simulink model "pid_pos"  (R2021a)
settings: Solver=ode5  StartTime=0.0  StopTime=15  MaxStep=0.001  RelTol=1e-3  EnableMultiTasking=on
values from neighbouring files (symbols this model uses):
  Kd = 0.158    [my_real_pendulum.m]
  Kd_phi = 0.22    [my_real_pendulum.m]
  Ki = 0.136    [my_real_pendulum.m]
  Kp = 0.522    [my_real_pendulum.m]
undefined symbols (not defined in the file or in its folder): Humusoft, MF624
libraries: sldrtlib x3, slpidlib x2, simulink x2
settings Model: Creator=fuka  LastModifiedBy=koubajac
settings SolverCC: AlgebraicLoopSolver=TrustRegion
settings DataIOCC: LimitDataPoints=on  SaveFormat=Array  SignalLoggingSaveFormat=ModelDataLogs  ReturnWorkspaceOutputs=off
settings OptimizationCC: ExpressionDepthLimit=2147483647  InitFltsAndDblsToZero=on
settings DebuggingCC: SaveWithParameterizedLinksMsg=none  UnderspecifiedInitializationDetection=Classic  MergeDetectMultiDrivingBlocksExec=none  SignalResolutionControl=TryResolveAllWithWarning  SolverPrmCheckMsg=warning  MultiTaskDSMMsg=warning  MultiTaskCondExecSysMsg=none  FcnCallInpInsideContextMsg=warning  StateNameClashWarn=warning  SFUnexpectedBacktrackingDiag=warning  SFNoUnconditionalDefaultTransitionDiag=warning  SFExecutionAtInitializationDiag=none  SFMachineParentedDataDiag=warning  ArithmeticOperatorsInVariantConditions=warning
settings ModelReferenceCC: PropagateSignalLabelsOutOfModel=off
settings SFSimCC: SimUseLocalCustomCode=off  CustomCodeUndefinedFunction=UseInterfaceOnly
settings RTWCC: Description=Simulink Desktop Real-Time  SystemTargetFile=sldrt.tlc  TemplateMakefile=sldrt.tmf  RTWUseLocalCustomCode=off  RTWCompilerOptimization=on
settings CodeAppCC: MaxIdLength=95  StateflowObjectComments=on
settings SimulinkDesktopRealTimeCC: TargetPreCompLibLocation=C:\MATLAB\R2021a\toolbox\sldrt\lib\win64  TargetLangStandard=C89/C90 (ANSI)
settings ConfigComp: CovMetricSettings=dw  CovSaveCumulativeToWorkspaceVar=on  CovSaveSingleToWorkspaceVar=on  CovExternalEMLEnable=off  CovSFcnEnable=off

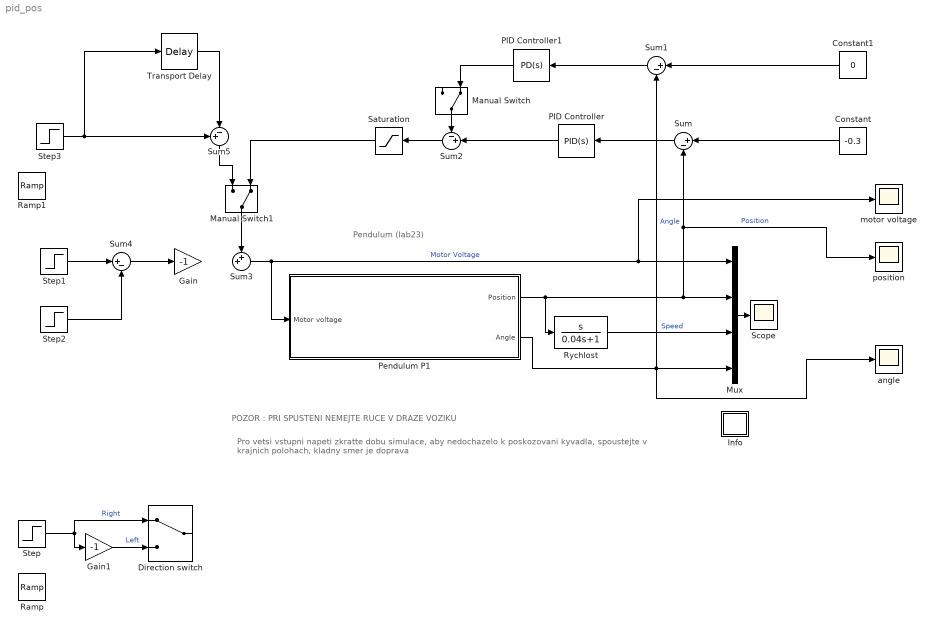
== system pid_pos ==
  note: POZOR : PRI SPUSTENI NEMEJTE RUCE V DRAZE VOZIKU
  note: Pro vetsi vstupni napeti zkratte dobu simulace, aby nedochazelo k poskozovani
      |  kyvadla, spoustejte v krajnich polohach, kladny smer je doprava
  note: Pendulum (lab23)
  Constant : Constant  Value=-0.3
  Constant1 : Constant  Value=0
  Direction switch : ManualSwitch
  Gain : Gain  Gain=-1
  Gain1 : Gain  Gain=-1
  Info : Subsystem
      mask Display: disp('?')
  Manual Switch : ManualSwitch  CurrentSetting=0
  Manual Switch1 : ManualSwitch  CurrentSetting=0
  Mux : Mux
  PID Controller : slpidlib/PID Controller  Controller=PID  Form=Parallel  TimeDomain=Continuous-time  UseExternalTs=off  SampleTime=-1  IntegratorMethod=Forward Euler  FilterMethod=Forward Euler  ControllerParametersSource=internal  P=Kp  I=Ki  D=Kd  UseFilter=on  N=100  TunerSelectOption=Transfer Function Based (PID Tuner App)  InitialConditionSource=internal  InitialConditionForIntegrator=0  InitialConditionForFilter=0  DifferentiatorICPrevScaledInput=0  ExternalReset=none  TrackingMode=off  Kt=1  LimitOutput=on  SatLimitsSource=internal  UpperSaturationLimit=1  LowerSaturationLimit=-1  LinearizeAsGain=on  AntiWindupMode=clamping  Kb=1  POutMin=[]  POutMax=[]  IOutMin=[]  IOutMax=[]  DOutMin=[]  DOutMax=[]  NOutMin=[]  NOutMax=[]  SumOutMin=[]  SumOutMax=[]  SaturationOutMin=[]  SaturationOutMax=[]  PParamMin=[]  PParamMax=[]  IParamMin=[]  IParamMax=[]  DParamMin=[]  DParamMax=[]  NParamMin=[]  NParamMax=[]  KbParamMin=[]  KbParamMax=[]  KtParamMin=[]  KtParamMax=[]  KbOutMin=[]  KbOutMax=[]  KtOutMin=[]  KtOutMax=[]  IntegratorOutMin=[]  IntegratorOutMax=[]  FilterOutMin=[]  FilterOutMax=[]  SumI1OutMin=[]  SumI1OutMax=[]  SumI2OutMin=[]  SumI2OutMax=[]  SumI3OutMin=[]  SumI3OutMax=[]  SumI4OutMin=[]  SumI4OutMax=[]  SumDOutMin=[]  SumDOutMax=[]  DifferentiatorOutMin=[]  DifferentiatorOutMax=[]  FilterDiffOutCoefMin=[]  FilterDiffOutCoefMax=[]  ReciprocalOutMin=[]  ReciprocalOutMax=[]  SumDenOutMin=[]  SumDenOutMax=[]  SumNumOutMin=[]  SumNumOutMax=[]  DivideOutMin=[]  DivideOutMax=[]  UdiffTsProdOutMin=[]  UdiffTsProdOutMax=[]  NTsProdOutMin=[]  NTsProdOutMax=[]  UintegralTsProdOutMin=[]  UintegralTsProdOutMax=[]  UngainTsProdOutMin=[]  UngainTsProdOutMax=[]  IntegratorContinuousStateAttributes=''  IntegratorStateMustResolveToSignalObject=off  IntegratorRTWStateStorageClass=Auto  FilterContinuousStateAttributes=''  FilterStateMustResolveToSignalObject=off  FilterRTWStateStorageClass=Auto  ParallelPVariant=InternalParameters  IdealPVariant=Disabled  IVariant=InternalParameters  DVariant=InternalParameters  IntegratorVariant=Continuous  SatVariant=Enabled  AWVariant=ContClampingParallel  PCopyVariant=Disabled  TRVariant=Disabled  FdbkBlocksVariant=Forward  IdealPFdbkVariant=Disabled  SatFdbkVariant=Disabled  DerivativeFilterVariant=ContFilter  NVariant=InternalParameters  NCopyVariant=Disabled  FilterICVariant=InternalICsFilter  IntegratorICVariant=InternalICs  ExternalResetVariant=Disabled  TRSumVariant=Passthrough  SumFdbkVariant=Disabled  SumVariant=Sum_PID  TsampFilterVariant=InternalTs  TsampNgainVariant=Passthrough  TsampIntegralVariant=Passthrough  ExternalSaturationOutDataTypeStr=Inherit: Same as second input
  PID Controller1 : slpidlib/PID Controller  Controller=PD  Form=Parallel  TimeDomain=Continuous-time  UseExternalTs=off  SampleTime=-1  IntegratorMethod=Forward Euler  FilterMethod=Forward Euler  ControllerParametersSource=internal  P=0  I=1  D=Kd_phi  UseFilter=on  N=100  TunerSelectOption=Transfer Function Based (PID Tuner App)  InitialConditionSource=internal  InitialConditionForIntegrator=0  InitialConditionForFilter=0  DifferentiatorICPrevScaledInput=0  ExternalReset=none  TrackingMode=off  Kt=1  LimitOutput=off  SatLimitsSource=internal  UpperSaturationLimit=inf  LowerSaturationLimit=-inf  LinearizeAsGain=on  AntiWindupMode=none  Kb=1  POutMin=[]  POutMax=[]  IOutMin=[]  IOutMax=[]  DOutMin=[]  DOutMax=[]  NOutMin=[]  NOutMax=[]  SumOutMin=[]  SumOutMax=[]  SaturationOutMin=[]  SaturationOutMax=[]  PParamMin=[]  PParamMax=[]  IParamMin=[]  IParamMax=[]  DParamMin=[]  DParamMax=[]  NParamMin=[]  NParamMax=[]  KbParamMin=[]  KbParamMax=[]  KtParamMin=[]  KtParamMax=[]  KbOutMin=[]  KbOutMax=[]  KtOutMin=[]  KtOutMax=[]  IntegratorOutMin=[]  IntegratorOutMax=[]  FilterOutMin=[]  FilterOutMax=[]  SumI1OutMin=[]  SumI1OutMax=[]  SumI2OutMin=[]  SumI2OutMax=[]  SumI3OutMin=[]  SumI3OutMax=[]  SumI4OutMin=[]  SumI4OutMax=[]  SumDOutMin=[]  SumDOutMax=[]  DifferentiatorOutMin=[]  DifferentiatorOutMax=[]  FilterDiffOutCoefMin=[]  FilterDiffOutCoefMax=[]  ReciprocalOutMin=[]  ReciprocalOutMax=[]  SumDenOutMin=[]  SumDenOutMax=[]  SumNumOutMin=[]  SumNumOutMax=[]  DivideOutMin=[]  DivideOutMax=[]  UdiffTsProdOutMin=[]  UdiffTsProdOutMax=[]  NTsProdOutMin=[]  NTsProdOutMax=[]  UintegralTsProdOutMin=[]  UintegralTsProdOutMax=[]  UngainTsProdOutMin=[]  UngainTsProdOutMax=[]  IntegratorContinuousStateAttributes=''  IntegratorStateMustResolveToSignalObject=off  IntegratorRTWStateStorageClass=Auto  FilterContinuousStateAttributes=''  FilterStateMustResolveToSignalObject=off  FilterRTWStateStorageClass=Auto  ParallelPVariant=InternalParameters  IdealPVariant=Disabled  IVariant=Disabled  DVariant=InternalParameters  IntegratorVariant=Disabled  SatVariant=Disabled  AWVariant=Disabled  PCopyVariant=Disabled  TRVariant=Disabled  FdbkBlocksVariant=Forward  IdealPFdbkVariant=Disabled  SatFdbkVariant=Disabled  DerivativeFilterVariant=ContFilter  NVariant=InternalParameters  NCopyVariant=Disabled  FilterICVariant=InternalICsFilter  IntegratorICVariant=Disabled  ExternalResetVariant=Disabled  TRSumVariant=Passthrough  SumFdbkVariant=Disabled  SumVariant=Sum_PD  TsampFilterVariant=InternalTs  TsampNgainVariant=Passthrough  TsampIntegralVariant=Disabled_SignalSpec  ExternalSaturationOutDataTypeStr=Inherit: Same as second input
  Pendulum P1 : Subsystem  InitFcn=warning off;  mask(Pendulum P1 in laboratory K23){Ts=0.001}
      mask prompts: Ts "Sampling time  {Ts = 0.001 s;   0.001 - 0.01 s}"
      mask help: Pendulum P1 in laboratory K23 - Real Time Communication
      mask Help:
      | Servo AMIRA S1, S4 in laboratory K23, K26 - Real Time Communication. <br><br>
      | 
      | This is a model of the Servomechanism, which is composed of two identical motors (motor and generator) connected together with solid motor shaft. First motor is used as a generator - it can be used to simulation of a varying  moment of inertia. The second motor takes control of the rotational speed of the servomechanism or the angle of turning of the motor shaft.<br>
      | 
      | There are two inputs and three outputs in the model. Inputs are voltages of generator and motor.
      | Outputs are speed of the servomechanism, the angle of turning of the motor shaft and current of the motor.<br><br>
      | In Simulink, the signals are normalized.
      mask Display: image(imread('P1pic.tif'))
  Ramp : simulink/Sources/Ramp  slope=1  start=0  InitialOutput=0
  Ramp1 : simulink/Sources/Ramp  slope=0.01  start=0  InitialOutput=0
  Rychlost : TransferFcn  Numerator=[1 0]  Denominator=[0.04 1]
  Saturation : Saturate  UpperLimit=1  LowerLimit=-1
  Scope : Scope
  Step : Step  After=0.35  SampleTime=0
  Step1 : Step  Time=0  After=0.3  SampleTime=0
  Step2 : Step  Time=2  After=0.3  SampleTime=0
  Step3 : Step  After=-0.4  SampleTime=0
  Sum : Sum  Inputs=|+-
  Sum1 : Sum  Inputs=|+-
  Sum2 : Sum  Inputs=-+|
  Sum3 : Sum  Inputs=++|
  Sum4 : Sum  Inputs=|+-
  Sum5 : Sum  Inputs=+-|
  Transport Delay : TransportDelay  DelayTime=1.6
  angle : Scope
  motor voltage : Scope
  position : Scope
  wires:
  Mux/1 -> Scope/1
  Pendulum P1/1(Position) -> Rychlost/1, position/1, Sum/2, Mux/2  "Position"
  Rychlost/1 -> Mux/3  "Speed"
  Pendulum P1/2(Angle) -> Mux/4, angle/1, Sum1/2  "Angle"
  Gain1/1 -> Direction switch/2  "Left"
  Step/1 -> Direction switch/1, Gain1/1  "Right"
  Sum/1 -> PID Controller/1
  Constant/1 -> Sum/1
  Constant1/1 -> Sum1/1
  PID Controller/1 -> Sum2/2
  Manual Switch/1 -> Sum2/1
  PID Controller1/1 -> Manual Switch/2
  Sum1/1 -> PID Controller1/1
  Sum3/1 -> motor voltage/1, Mux/1, Pendulum P1/1(Motor voltage)  "Motor Voltage"
  Manual Switch1/1 -> Sum3/1
  Sum4/1 -> Gain/1
  Step1/1 -> Sum4/1
  Step2/1 -> Sum4/2
  Sum5/1 -> Manual Switch1/1
  Transport Delay/1 -> Sum5/2
  Step3/1 -> Transport Delay/1, Sum5/1
  Sum2/1 -> Saturation/1
  Saturation/1 -> Manual Switch1/2

== system pid_pos/Info ==
  note: Urceno pro mereni prechodovych charakteristik realneho systemu inverzni kyvadlo.
      |  Periodu vzorkovani Ts volte v rozsahu 0.0005 s < Ts < 0.001 s  (dop. Ts = 0.001 s).
  note: Vozik presunte do leve krajni polohy. Po spusteni simulace dojede k prave krajni
      | poloze. Presunte jej ke koncovemu spinaci a zmente znamenko zesileni. Vozik
      | se vrati do vychozi polohy. Pri vetsim vstupnim napeti zkratte dobu simulace!!!
  note: Umisteni voziku
  note: Merena data jsou ukladana po radcich do matice ty v pracovnim prostoru Matlabu.
      | Prvni sloupec matice ty predstavuje cas a dalsi pak jednotlive promenne v poradi
      | vstupu do bloku multiplexoru osciloskopu. Krome toho je jeste k dispozici samotny
      | vektor casu tout. Prubehy velicin zobrazite napr. prikazem: plot(ty(:,1),ty(:,2:4)).
  note: Nezapomente si ulozit namerena data napr. prikazem: save <jmeno> ty
  note: Ve formatu ASCII je pak ulozite prikazem: save <jmeno> ty -ascii
  note: C: J.Fuka 2007-2015 pro Matlab 2014b s RTWT
  note: Kyvadlo P1 (lab. 23)

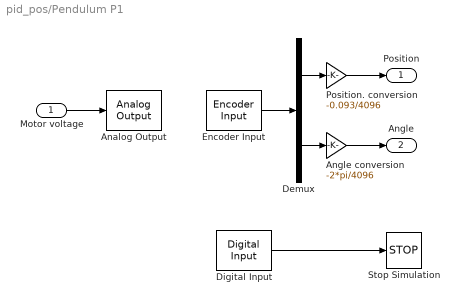
== system pid_pos/Pendulum P1 ==
  Motor voltage : Inport
  Analog Output : sldrtlib/Analog Output  SampleTime=Ts  MaxMissedTicks=200  ShowMissedTicks=off  YieldWhenWaiting=on  DrvName=Humusoft/MF624  DrvAddress=4294967295  DrvOptions=0  Channels=1  RangeMode=2  VoltRange=1  InitialValue=0  FinalValue=0
      settings: AttributesFormatString=Humusoft\nMF624 [auto]
  Angle conversion : Gain  Gain=-2*pi/4096
  Demux : Demux  Outputs=2
      settings: DisplayOption=none
  Digital Input : sldrtlib/Digital Input  SampleTime=0.005  MaxMissedTicks=100  ShowMissedTicks=off  YieldWhenWaiting=off  DrvName=Humusoft/MF624  DrvAddress=4294967295  DrvOptions=0  Channels=3  BitMode=1  DataType=9
      settings: AttributesFormatString=Humusoft\nMF624 [auto]  SourceProductBaseCode=WT
  Encoder Input : sldrtlib/Encoder Input  SampleTime=Ts  MaxMissedTicks=200  ShowMissedTicks=off  YieldWhenWaiting=on  DrvName=Humusoft/MF624  DrvAddress=4294967295  DrvOptions=0  Channels=[1 2]  QuadMode=3  IndexPulse=2  InputFilter=Inf  DataType=1
      settings: AttributesFormatString=Humusoft\nMF624 [auto]
  Position. conversion : Gain  Gain=-0.093/4096
  Stop Simulation : Stop
  Position : Outport
  Angle : Outport  Port=2
  wires:
  Position. conversion/1 -> Position/1
  Demux/2 -> Angle conversion/1
  Angle conversion/1 -> Angle/1
  Encoder Input/1 -> Demux/1
  Demux/1 -> Position. conversion/1
  Digital Input/1 -> Stop Simulation/1
  Motor voltage/1 -> Analog Output/1
